simulink model "lab02es3"  (R2021b)
settings: Solver=VariableStepAuto  StartTime=0.0  StopTime=1000  RelTol=1e-3
undefined symbols (not defined in the file): entity, entitySys, exprnd, m, n, ShowAttr
settings Model: Creator=francescafornasier  LastModifiedBy=francescafornasier

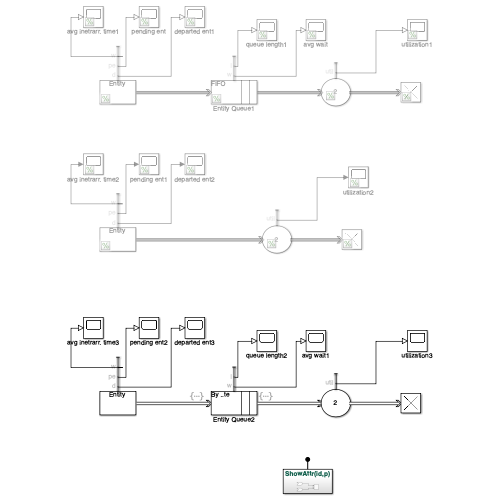
[thumbnail: Simulink's stored preview of the top-level diagram]
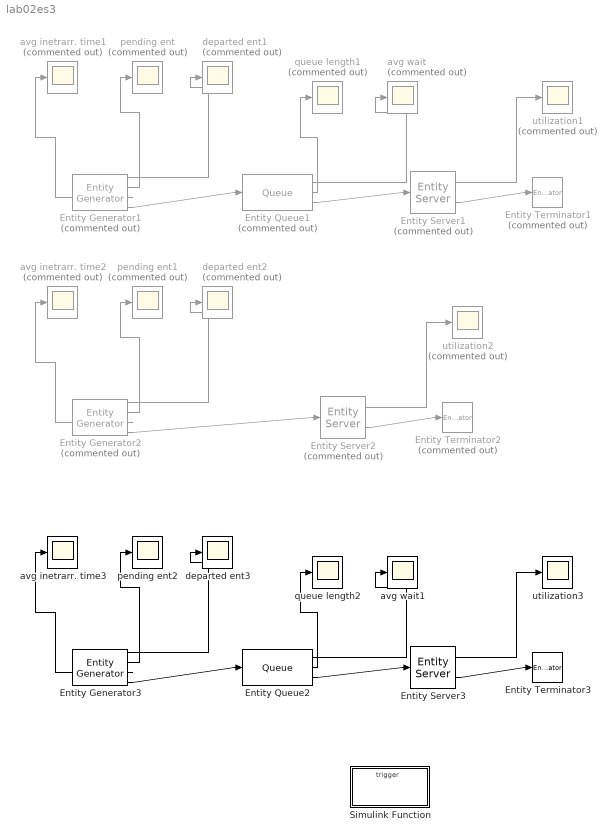
== system lab02es3 ==
  Entity Generator1 : EntityGenerator  Commented=on  OutputPortMessageModes=n,n,n,m  TimeSource=MATLAB action  IntergenerationTimeAction=dt = exprnd(1);  GenerateEntityAtSimulationStart=off  NumberEntitiesDeparted=on  PendingEntityInBlock=on  AverageIntergenerationTime=on  EntityType=Structured  EntityTypeName=Entity
      settings: OutputPortMap=o0,o1,o2,o3
  Entity Generator2 : EntityGenerator  Commented=on  OutputPortMessageModes=n,n,n,m  TimeSource=MATLAB action  IntergenerationTimeAction=dt = exprnd(1);  GenerateEntityAtSimulationStart=off  NumberEntitiesDeparted=on  PendingEntityInBlock=on  AverageIntergenerationTime=on  EntityType=Structured  EntityTypeName=Entity
      settings: OutputPortMap=o0,o1,o2,o3
  Entity Generator3 : EntityGenerator  OutputPortMessageModes=n,n,n,m  TimeSource=MATLAB action  IntergenerationTimeAction=dt = exprnd(1);  GenerateEntityAtSimulationStart=off  AttributeName=PriorityAttribute  NumberEntitiesDeparted=on  PendingEntityInBlock=on  AverageIntergenerationTime=on  EntityType=Structured  EntityTypeName=Entity
      settings: OutputPortMap=o0,o1,o2,o3
  Entity Queue1 : Queue  Commented=on  InputPortMessageModes=m  OutputPortMessageModes=n,n,m  Capacity=5  AverageWait=on  AverageQueueLength=on
      settings: OutputPortMap=o2,o3,o5
  Entity Queue2 : Queue  InputPortMessageModes=m  OutputPortMessageModes=n,n,m  Capacity=5  QueueType=Priority  EntryAction=entity.PriorityAttribute = randi([1,2],1,1)  ExitAction=ShowAttr(entitySys.id,entity.PriorityAttribute)  AverageWait=on  AverageQueueLength=on
      settings: OutputPortMap=o2,o3,o5
  Entity Server1 : EntityServer  Commented=on  InputPortMessageModes=m  OutputPortMessageModes=n,m  Capacity=2  ServiceTimeSource=MATLAB action  ServiceTimeValue=exprnd(1)  ServiceTimeAction=dt = exprnd(1);  Utilization=on
      settings: OutputPortMap=o5,o9
  Entity Server2 : EntityServer  Commented=on  InputPortMessageModes=m  OutputPortMessageModes=n,m  Capacity=2  ServiceTimeSource=MATLAB action  ServiceTimeValue=exprnd(1)  ServiceTimeAction=dt = exprnd(1);  Utilization=on
      settings: OutputPortMap=o5,o9
  Entity Server3 : EntityServer  InputPortMessageModes=m  OutputPortMessageModes=n,m  Capacity=2  ServiceTimeSource=MATLAB action  ServiceTimeValue=exprnd(1)  ServiceTimeAction=dt = exprnd(1);  Utilization=on
      settings: OutputPortMap=o5,o9
  Entity Terminator1 : EntityTerminator  Commented=on  InputPortMessageModes=m
  Entity Terminator2 : EntityTerminator  Commented=on  InputPortMessageModes=m
  Entity Terminator3 : EntityTerminator  InputPortMessageModes=m
  Simulink Function : Subsystem  TreatAsAtomicUnit=on
  avg inetrarr. time1 : Scope  Commented=on
  avg inetrarr. time2 : Scope  Commented=on
  avg inetrarr. time3 : Scope
  avg wait : Scope  Commented=on
  avg wait1 : Scope
  departed ent1 : Scope  Commented=on
  departed ent2 : Scope  Commented=on
  departed ent3 : Scope
  pending ent : Scope  Commented=on
  pending ent1 : Scope  Commented=on
  pending ent2 : Scope
  queue length1 : Scope  Commented=on
  queue length2 : Scope
  utilization1 : Scope  Commented=on
  utilization2 : Scope  Commented=on
  utilization3 : Scope
  wires:
  Entity Server1/1 -> utilization1/1
  Entity Generator1/3 -> avg inetrarr. time1/1
  Entity Queue1/2 -> queue length1/1
  Entity Generator1/4 -> Entity Queue1/1
  Entity Generator1/1 -> departed ent1/1
  Entity Generator1/2 -> pending ent/1
  Entity Server1/2 -> Entity Terminator1/1
  Entity Queue1/3 -> Entity Server1/1
  Entity Queue1/1 -> avg wait/1
  Entity Server2/2 -> Entity Terminator2/1
  Entity Generator2/2 -> pending ent1/1
  Entity Generator2/1 -> departed ent2/1
  Entity Generator2/3 -> avg inetrarr. time2/1
  Entity Generator2/4 -> Entity Server2/1
  Entity Server2/1 -> utilization2/1
  Entity Generator3/4 -> Entity Queue2/1
  Entity Server3/2 -> Entity Terminator3/1
  Entity Generator3/2 -> pending ent2/1
  Entity Generator3/1 -> departed ent3/1
  Entity Generator3/3 -> avg inetrarr. time3/1
  Entity Queue2/2 -> queue length2/1
  Entity Queue2/3 -> Entity Server3/1
  Entity Server3/1 -> utilization3/1
  Entity Queue2/1 -> avg wait1/1

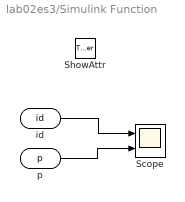
== system lab02es3/Simulink Function ==
  ShowAttr : TriggerPort  TriggerType=function-call  IsSimulinkFunction=on  FunctionName=ShowAttr  FunctionVisibility=scoped  VariantControl=(inherit)
  Scope : Scope  NumInputPorts=2
  id : ArgIn  DisableCoverage=on  ArgumentName=id
  p : ArgIn  DisableCoverage=on  Port=2  ArgumentName=p
  wires:
  id/1 -> Scope/1
  p/1 -> Scope/2
